simulink model "TEMA_HMA_WMA_TB"  (R2024a)
settings: Solver=VariableStepAuto  StartTime=0.0  StopTime=700  RelTol=1e-3
PreLoadFcn:
  | N = 100;
libraries: dspstat3 x5, dspsrcs4 x1
settings Model: Creator=kschutz  LastModifiedBy=kschutz
settings SolverCC: AlgebraicLoopSolver=TrustRegion
settings OptimizationCC: DefaultParameterBehavior=Inlined  EnhancedBackFolding=on  PassReuseOutputArgsAs=Individual arguments  ZeroExternalMemoryAtStartup=off  ZeroInternalMemoryAtStartup=off  OptimizeBlockOrder=speed  DifferentSizesBufferReuse=on  OptimizationCustomize=off  EfficientTunableParamExpr=on
settings DebuggingCC: ParameterTunabilityLossMsg=error  UnconnectedInputMsg=warning  UnconnectedOutputMsg=warning  UnconnectedLineMsg=warning
settings ModelReferenceCC: EnableRefExpFcnMdlSchedulingChecks=on
settings SFSimCC: MATLABDynamicMemAlloc=off
settings RTWCC: Description=Embedded Coder  SystemTargetFile=ert.tlc  GenCodeOnly=on  TemplateMakefile=ert_default_tmf  GenerateReport=on  LaunchReport=on  GenerateWebview=on  GPUComputeCapability=3.5  DLArmComputeVersion=19.05
settings CodeAppCC: ForceParamTrailComments=on  IgnoreCustomStorageClasses=off  OperatorAnnotations=on  SimulinkDataObjDesc=on  SFDataObjDesc=on  InsertBlockDesc=on
settings ERTTargetCC: TargetLangStandard=C99 (ISO)  GenerateSampleERTMain=on  InlinedParameterPlacement=NonHierarchical  ERTCustomFileTemplate=example_file_process.tlc

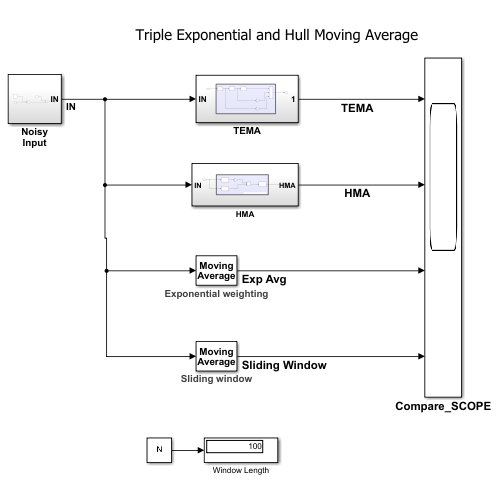
[thumbnail: Simulink's stored preview of the top-level diagram]
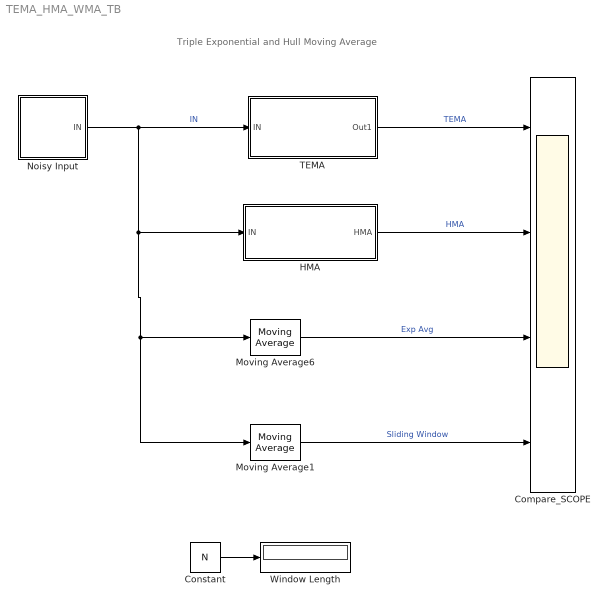
== system TEMA_HMA_WMA_TB ==
  note: Triple Exponential and Hull Moving Average
  Compare_SCOPE : Scope  NumInputPorts=4
  Constant : Constant  Value=N
  HMA : Subsystem
  Moving Average1 : dspstat3/Moving Average  Method=Sliding window  ForgettingFactorPort=off  SpecifyWindowLength=on  WindowLength=N  OverlapLength=N-1  AllowArbitraryInputLength=off  ForgettingFactor=(N-1)/N  SimulateUsing=Interpreted execution
      settings: AttributesFormatString=%<Method>
  Moving Average6 : dspstat3/Moving Average  Method=Exponential weighting  ForgettingFactorPort=off  SpecifyWindowLength=on  WindowLength=20  OverlapLength=19  AllowArbitraryInputLength=off  ForgettingFactor=(N-1)/N  SimulateUsing=Interpreted execution
      settings: AttributesFormatString=%<Method>
  Noisy Input : Subsystem
  TEMA : Subsystem
  Window Length : Display
  wires:
  TEMA/1(Out1) -> Compare_SCOPE/1  "TEMA"
  Constant/1 -> Window Length/1
  Noisy Input/1(IN) -> TEMA/1(IN), HMA/1(IN), Moving Average6/1, Moving Average1/1  "IN"
  HMA/1(HMA) -> Compare_SCOPE/2  "HMA"
  Moving Average1/1 -> Compare_SCOPE/4  "Sliding Window"
  Moving Average6/1 -> Compare_SCOPE/3  "Exp Avg"

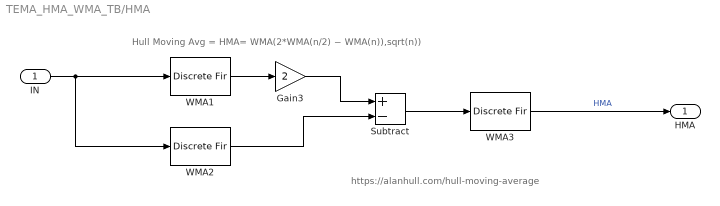
== system TEMA_HMA_WMA_TB/HMA ==
  note: https://alanhull.com/hull-moving-average
  note: Hull Moving Avg = HMA= WMA(2*WMA(n/2) − WMA(n)),sqrt(n))
  IN : Inport
  Gain3 : Gain  Gain=2
  Subtract : Sum  Inputs=+-
  WMA1 : DiscreteFir  Coefficients=[N/2:-1:1]/sum(1:N/2)
  WMA2 : DiscreteFir  Coefficients=[N:-1:1]/sum(1:N)
  WMA3 : DiscreteFir  Coefficients=[sqrt(N):-1:1]/sum(1:sqrt(N))
  HMA : Outport
  wires:
  Subtract/1 -> WMA3/1
  WMA2/1 -> Subtract/2
  IN/1 -> WMA2/1, WMA1/1
  Gain3/1 -> Subtract/1
  WMA1/1 -> Gain3/1
  WMA3/1 -> HMA/1  "HMA"

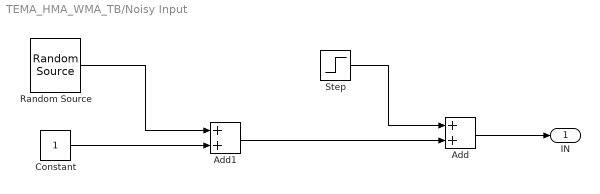
== system TEMA_HMA_WMA_TB/Noisy Input ==
  Add : Sum
  Add1 : Sum
  Constant : Constant  SampleTime=1
  Random Source : dspsrcs4/Random Source  SrcType=Gaussian  MinVal=0  MaxVal=1  MeanVal=0  VarVal=.2  RepMode=Specify seed  rawSeed=123  IsInherit=off  SampTime=1  SampFrame=1  OutComplex=Real  DataType=double  SimulateUsing=Interpreted execution
  Step : Step  Time=500  SampleTime=0
  IN : Outport  VectorParamsAs1DForOutWhenUnconnected=off
  wires:
  Constant/1 -> Add1/2
  Random Source/1 -> Add1/1
  Add/1 -> IN/1
  Add1/1 -> Add/2
  Step/1 -> Add/1

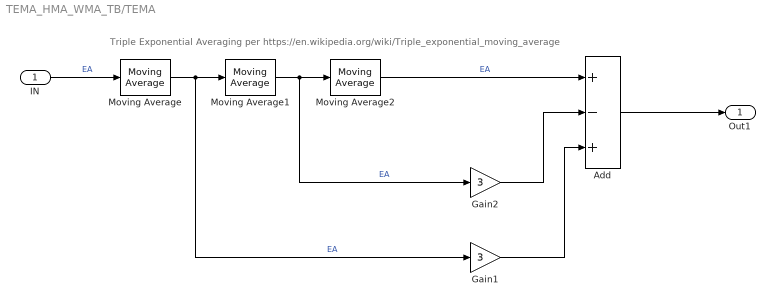
== system TEMA_HMA_WMA_TB/TEMA ==
  note: Triple Exponential Averaging per https://en.wikipedia.org/wiki/Triple_exponential_moving_average
  IN : Inport
  Add : Sum  Inputs=+-+
  Gain1 : Gain  Gain=3
  Gain2 : Gain  Gain=3
  Moving Average : dspstat3/Moving Average  Method=Exponential weighting  ForgettingFactorPort=off  SpecifyWindowLength=on  WindowLength=20  OverlapLength=19  AllowArbitraryInputLength=off  ForgettingFactor=(N-1)/N  SimulateUsing=Interpreted execution
      settings: AttributesFormatString=FF = %<ForgettingFactor>
  Moving Average1 : dspstat3/Moving Average  Method=Exponential weighting  ForgettingFactorPort=off  SpecifyWindowLength=on  WindowLength=20  OverlapLength=19  AllowArbitraryInputLength=off  ForgettingFactor=(N-1)/N  SimulateUsing=Interpreted execution
      settings: AttributesFormatString=FF = %<ForgettingFactor>
  Moving Average2 : dspstat3/Moving Average  Method=Exponential weighting  ForgettingFactorPort=off  SpecifyWindowLength=on  WindowLength=20  OverlapLength=19  AllowArbitraryInputLength=off  ForgettingFactor=(N-1)/N  SimulateUsing=Interpreted execution
      settings: AttributesFormatString=FF = %<ForgettingFactor>
  Out1 : Outport
  wires:
  Moving Average/1 -> Gain1/1, Moving Average1/1  "EA"
  Moving Average2/1 -> Add/1  "EA"
  Gain2/1 -> Add/2
  Gain1/1 -> Add/3
  IN/1 -> Moving Average/1  "EA"
  Moving Average1/1 -> Gain2/1, Moving Average2/1  "EA"
  Add/1 -> Out1/1
